simulink model "single_phase_full_H_bridge_inverter"  (R2018a)
settings: Solver=VariableStepAuto  StartTime=0.0  StopTime=10  RelTol=1e-3
libraries: powerlib x12
settings Model: EnablePacing=on  Creator=Asus  LastModifiedBy=Asus

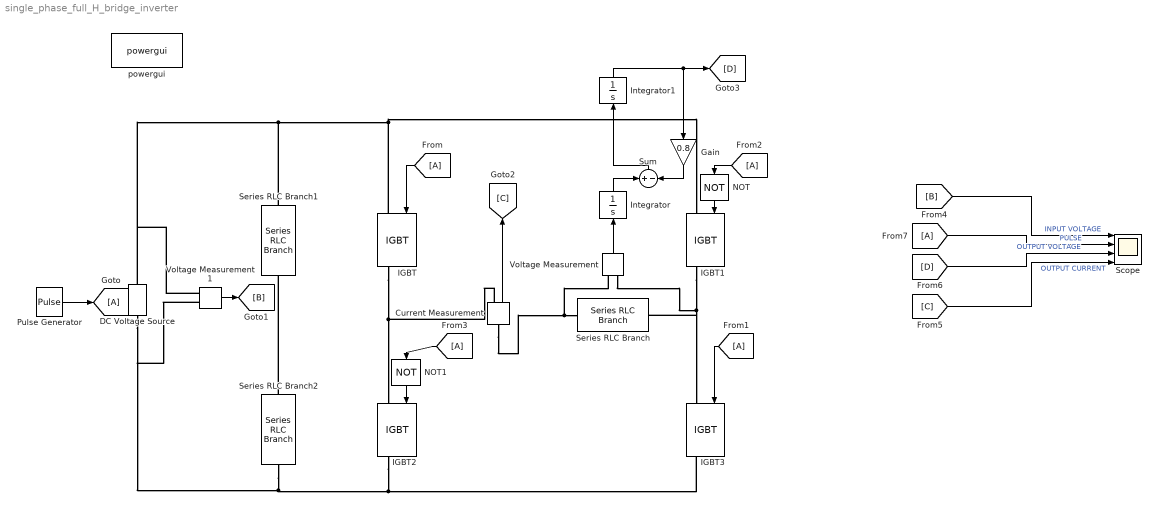
== system single_phase_full_H_bridge_inverter ==
  Current Measurement : powerlib/Measurements/Current Measurement  PhasorSimulation=off  OutputType=Complex  PSBequivalent=0
  DC Voltage Source : powerlib/Electrical Sources/DC Voltage Source  Amplitude=100  Measurements=None
  Gain : Gain  Gain=0.8
  IGBT{,1..3} (4 alike) : powerlib/Power Electronics/IGBT  Ron=0.001  Lon=0  Vf=1  Tf=1e-6  Tt=2e-6  IC=0  Rs=1e5  Cs=inf  Measurements=on
  Integrator : Integrator
  Integrator1 : Integrator
  NOT : Logic  Operator=NOT  IconShape=distinctive  AllPortsSameDT=off  OutDataTypeStr=boolean
  NOT1 : Logic  Operator=NOT  IconShape=distinctive  AllPortsSameDT=off  OutDataTypeStr=boolean
  Pulse Generator : DiscretePulseGenerator  PulseType=Time based  Period=1  PulseWidth=50
  Scope : Scope  NumInputPorts=4
  Series RLC Branch : powerlib/Elements/Series RLC Branch  LConnTagsString=__new0  RConnTagsString=__new0  BranchType=Open circuit  Resistance=1e3  Inductance=1  SetiL0=off  InitialCurrent=0  Capacitance=1  Setx0=off  InitialVoltage=0  Measurements=None
  Series RLC Branch1 : powerlib/Elements/Series RLC Branch  LConnTagsString=__new0  RConnTagsString=__new0  BranchType=RC  Resistance=0.05  Inductance=0  SetiL0=off  InitialCurrent=0  Capacitance=1e-6  Setx0=off  InitialVoltage=0  Measurements=None
  Series RLC Branch2 : powerlib/Elements/Series RLC Branch  LConnTagsString=__new0  RConnTagsString=__new0  BranchType=RC  Resistance=0.05  Inductance=0  SetiL0=off  InitialCurrent=0  Capacitance=1e-6  Setx0=off  InitialVoltage=0  Measurements=None
  Sum : Sum  Inputs=+-
  Voltage Measurement : powerlib/Measurements/Voltage Measurement  PhasorSimulation=off  OutputType=Complex  PSBequivalent=0
  Voltage Measurement1 : powerlib/Measurements/Voltage Measurement  PhasorSimulation=off  OutputType=Complex  PSBequivalent=0
  powergui : powerlib/powergui  Priority=1  SimulationMode=Continuous  SampleTime=50e-6  frequency=60  Iterations=50  frequencyindice=0  Pbase=100e6  ErrMax=1e-4  UnitsV=kV  UnitsW=MW  buscounter=0  FunctionMessages=off  echomessages=off  EnableUseOfTLC=off  CurrentSourceSwitches=off  DisableSnubberDevices=off  DisableRonSwitches=off  DisableVfSwitches=off  DisplayEquations=off  SolverType=Tustin/Backward Euler (TBE)  Interpol=off  ExternalGateDelay=off  methode=off  Ts=100  x0status=blocks  SPID=on  SwTol=0  HookPort=off  RestoreLinks=warning  ResistiveCurrentMeasurement=off  Frange=[0:2:500]  Ylog=off  Xlog=on  ShowGrid=off  save=off  variable=ZData  structure=0  ZoomFFT=off  StartTime=0.0  cycles=1  DisplayStyle=1  fundamental=60  FreqAxis=off  MaxFrequency=1000  frequencyindicesteady=1  RmsSteady=1  display=off
  wires:
  Pulse Generator/1 -> [A]
  [A] -> IGBT/1
  [A] -> IGBT3/1
  NOT/1 -> IGBT1/1
  [A] -> NOT/1
  [A] -> NOT1/1
  NOT1/1 -> IGBT2/1
  Voltage Measurement1/1 -> [B]
  Current Measurement/1 -> [C]
  [D] -> Scope/3  "OUTPUT VOLTAGE"
  [B] -> Scope/1  "INPUT VOLTAGE"
  [C] -> Scope/4  "OUTPUT CURRENT"
  [A] -> Scope/2  "PULSE"
  Integrator1/1 -> [D], Gain/1
  Voltage Measurement/1 -> Integrator/1
  Sum/1 -> Integrator1/1
  Gain/1 -> Sum/2
  Integrator/1 -> Sum/1
  connections:
  IGBT2/RConn1 -- Voltage Measurement1/LConn2 -- DC Voltage Source/LConn1 -- Series RLC Branch2/RConn1 -- IGBT3/RConn1
  IGBT/LConn1 -- Voltage Measurement1/LConn1 -- DC Voltage Source/RConn1 -- Series RLC Branch1/LConn1 -- IGBT1/LConn1
  IGBT1/RConn1 -- Voltage Measurement/LConn2 -- Series RLC Branch/RConn1 -- IGBT3/LConn1
  IGBT/RConn1 -- Current Measurement/RConn1 -- IGBT2/LConn1
  Series RLC Branch2/LConn1 -- Series RLC Branch1/RConn1
  Current Measurement/LConn1 -- Voltage Measurement/LConn1 -- Series RLC Branch/LConn1
